simulink model "fuzzy_uirs"  (R2022a)
settings: Solver=FixedStepAuto  StartTime=0.0  StopTime=17  FixedStep=0.01  RelTol=1e-3
undefined symbols (not defined in the file): b, g, J, Ke, Kt, L, R
libraries: simulink_extras x9, slpidlib x3, fuzblock x3, simulink x1
settings Model: Creator=ngovi  LastModifiedBy=ngovi

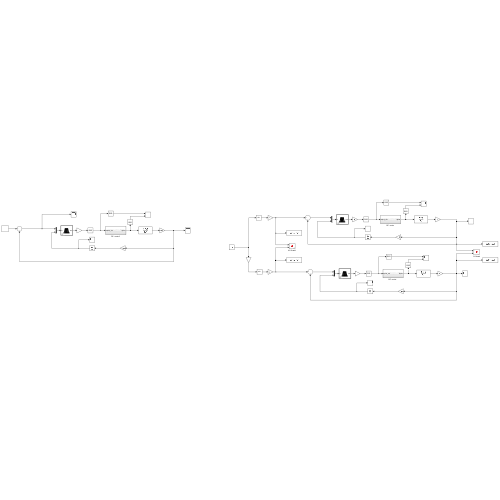
[thumbnail: Simulink's stored preview of the top-level diagram]
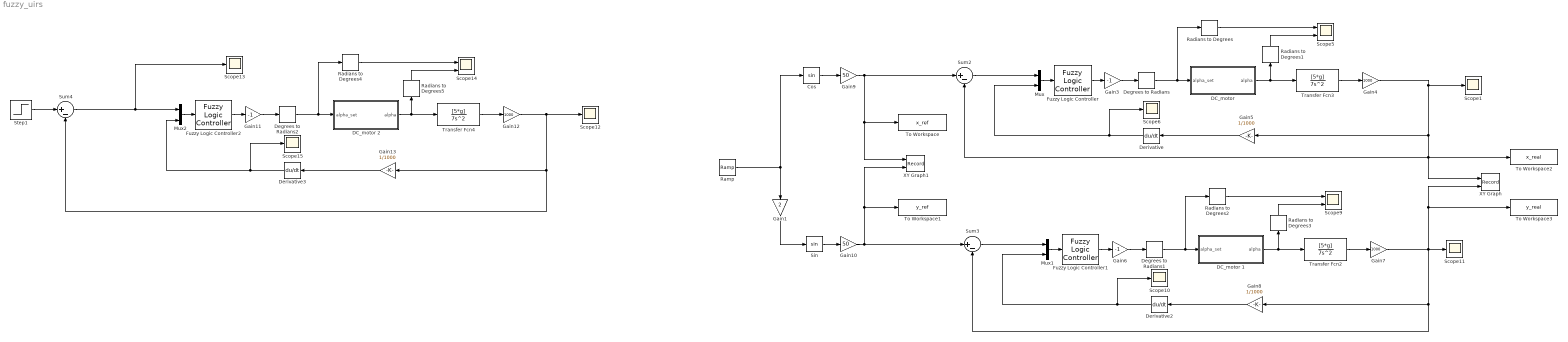
== system fuzzy_uirs ==
  Cos : Trigonometry
  "DC_motor " : Subsystem
  DC_motor 1 : Subsystem
  DC_motor 2 : Subsystem
  Degrees to Radians : simulink_extras/Transformations/Degrees to Radians
  Degrees to Radians1 : simulink_extras/Transformations/Degrees to Radians
  Degrees to Radians2 : simulink_extras/Transformations/Degrees to Radians
  Derivative : Derivative
  Derivative2 : Derivative
  Derivative3 : Derivative
  Fuzzy Logic Controller : fuzblock/Fuzzy Logic  Controller  FIS=logic3_3  OutputSampleNumber=101  DataType=double  FuzzifiedInputs=off  RuleFiringStrengths=off  RuleOutputs=off  AggregatedOutputs=off  SimulateUsing=Interpreted execution  OutOfRangeInputValueMessage=warning  NoRuleFiredMessage=warning  EmptyOutputFuzzySetMessage=warning
  Fuzzy Logic Controller1 : fuzblock/Fuzzy Logic  Controller  FIS=logic3_3  OutputSampleNumber=101  DataType=double  FuzzifiedInputs=off  RuleFiringStrengths=off  RuleOutputs=off  AggregatedOutputs=off  SimulateUsing=Interpreted execution  OutOfRangeInputValueMessage=warning  NoRuleFiredMessage=warning  EmptyOutputFuzzySetMessage=warning
  Fuzzy Logic Controller2 : fuzblock/Fuzzy Logic  Controller  FIS=logic3_3  OutputSampleNumber=101  DataType=double  FuzzifiedInputs=off  RuleFiringStrengths=off  RuleOutputs=off  AggregatedOutputs=off  SimulateUsing=Interpreted execution  OutOfRangeInputValueMessage=warning  NoRuleFiredMessage=warning  EmptyOutputFuzzySetMessage=warning
  Gain1 : Gain  Gain=2
  Gain10 : Gain  Gain=50
  Gain11 : Gain  Gain=-1
  Gain12 : Gain  Gain=1000
  Gain13 : Gain  Gain=1/1000
  Gain3 : Gain  Gain=-1
  Gain4 : Gain  Gain=1000
  Gain5 : Gain  Gain=1/1000
  Gain6 : Gain  Gain=-1
  Gain7 : Gain  Gain=1000
  Gain8 : Gain  Gain=1/1000
  Gain9 : Gain  Gain=50
  Mux : Mux  Inputs=2
  Mux1 : Mux  Inputs=2
  Mux2 : Mux  Inputs=2
  Radians to Degrees{,1..5} (6 alike) : simulink_extras/Transformations/Radians to Degrees
  Ramp : simulink/Sources/Ramp  slope=2*pi/15  start=0  InitialOutput=1
  Scope{1,6,10..13,15} (7 alike) : Scope
  Scope14 : Scope  NumInputPorts=2
  Scope5 : Scope  NumInputPorts=2
  Scope9 : Scope  NumInputPorts=2
  Sin : Trigonometry
  Step1 : Step  Time=0  After=50  SampleTime=0
  Sum2 : Sum  Inputs=|+-
  Sum3 : Sum  Inputs=|+-
  Sum4 : Sum  Inputs=|+-
  To Workspace : ToWorkspace  VariableName=x_ref  SampleTime=-1
  To Workspace1 : ToWorkspace  VariableName=y_ref  SampleTime=-1
  To Workspace2 : ToWorkspace  VariableName=x_real  SampleTime=-1
  To Workspace3 : ToWorkspace  VariableName=y_real  SampleTime=-1
  Transfer Fcn2 : TransferFcn  Numerator=[5*g]  Denominator=[7 0 0]
  Transfer Fcn3 : TransferFcn  Numerator=[5*g]  Denominator=[7 0 0]
  Transfer Fcn4 : TransferFcn  Numerator=[5*g]  Denominator=[7 0 0]
  XY Graph : Record  FileSettingsInternal="{\"entries\":[{\"content\":{\"excelSettings\":{\"content\":{},\"type\":\"Streamout.ExcelSettings\"}},\"type\":\"Streamout.FileSettingStorage\",\"uuid\":\"afb4c868-1969-4ea8-89d1-48caf8c4fd68\"}],\"packageUris\":[\"http://schema.mathworks.com/mf0/streamout_blocks/R2020a\"],\"version\":\"1.0\"}"  Layout=[1 1]  SignalsInternal="{\"entries\":[{\"content\":{\"signals\":[{\"content\":{\"blockPath\":[\"fuzzy_uirs/XY Graph\"],\"channel\":[],\"dimensions\":[1],\"domain\":\"fuzzy_uirs/XY Graph\",\"lineColor\":\"#a2142f\",\"plots\":[1],\"port\":1,\"sid\":[\"\"],\"signalID\":79152,\"signalName\":\"Gain4\"},\"type\":\"RecordBlkView.Signal\",\"uuid\":\"c0bbbc2e-870e-4cf8-b3f4-c9450fb1db15\"},{\"content\":{\"blockPath\":[\"fuzzy_uirs/XY Graph\"],\"channel\":[],\"dimensions\":[1],\"domain\":\"fuzzy_uirs/XY Graph\",\"lineColor\":\"#139fff\",\"plots\":[1],\"port\":2,\"sid\":[\"\"],\"signalID\":79156,\"signalName\":\"Gain7\"},\"type\":\"RecordBlkView.Signal\",\"uuid\":\"cc5d9cb4-a176-4346-b85d-aba7a873011e\"}]},\"type\":\"RecordBlkView.InputSignals\",\"uuid\":\"800058d3-d4f3-4397-acbe-427882f86b80\"}],\"packageUris\":[\"http://schema.mathworks.com/mf0/streamout_blocks/R2020a\"],\"version\":\"1.0\"}"  VisualizationBindings="{\"xyplotplugin\":{\"info\":[{\"series\":[{\"bindingParametersList\":[{\"parameter\":\"X-Axis\",\"signalID\":79152,\"signalName\":\"Gain4\"},{\"parameter\":\"Y-Axis\",\"signalID\":79156,\"signalName\":\"Gain7\"}],\"seriesID\":60483}],\"subplotID\":1}]}}"  CompatibilityTag=XY
  XY Graph1 : Record  FileSettingsInternal="{\"entries\":[{\"content\":{\"excelSettings\":{\"content\":{},\"type\":\"Streamout.ExcelSettings\"}},\"type\":\"Streamout.FileSettingStorage\",\"uuid\":\"2a686f37-4683-499c-9b28-704c226203bf\"}],\"packageUris\":[\"http://schema.mathworks.com/mf0/streamout_blocks/R2020a\"],\"version\":\"1.0\"}"  Layout=[1 1]  SignalsInternal="{\"entries\":[{\"content\":{\"signals\":[{\"content\":{\"blockPath\":[\"fuzzy_uirs/XY Graph1\"],\"channel\":[],\"dimensions\":[1],\"domain\":\"fuzzy_uirs/XY Graph1\",\"lineColor\":\"#a2142f\",\"plots\":[1],\"port\":1,\"sid\":[\"\"],\"signalID\":79160,\"signalName\":\"Gain9\"},\"type\":\"RecordBlkView.Signal\",\"uuid\":\"5bdc1996-2df4-4c65-8b97-25dc56d0c1d6\"},{\"content\":{\"blockPath\":[\"fuzzy_uirs/XY Graph1\"],\"channel\":[],\"dimensions\":[1],\"domain\":\"fuzzy_uirs/XY Graph1\",\"lineColor\":\"#139fff\",\"plots\":[1],\"port\":2,\"sid\":[\"\"],\"signalID\":79164,\"signalName\":\"Gain10\"},\"type\":\"RecordBlkView.Signal\",\"uuid\":\"afd1a10f-c0e4-4f62-abbc-f7fd10843523\"}]},\"type\":\"RecordBlkView.InputSignals\",\"uuid\":\"c62105ff-e949-4276-9948-db52a4e51b1c\"}],\"packageUris\":[\"http://schema.mathworks.com/mf0/streamout_blocks/R2020a\"],\"version\":\"1.0\"}"  VisualizationBindings="{\"xyplotplugin\":{\"info\":[{\"series\":[{\"bindingParametersList\":[{\"parameter\":\"X-Axis\",\"signalID\":79160,\"signalName\":\"Gain9\"},{\"parameter\":\"Y-Axis\",\"signalID\":79164,\"signalName\":\"Gain10\"}],\"seriesID\":17296}],\"subplotID\":1}]}}"  CompatibilityTag=XY
  wires:
  Fuzzy Logic Controller/1 -> Gain3/1
  Sum2/1 -> Mux/1
  "DC_motor "/1(alpha) -> Transfer Fcn3/1, Radians to Degrees1/1
  Mux/1 -> Fuzzy Logic Controller/1
  Derivative/1 -> Mux/2, Scope6/1
  Gain3/1 -> Degrees to Radians/1
  Degrees to Radians/1 -> Radians to Degrees/1, "DC_motor "/1(alpha_set)
  Transfer Fcn3/1 -> Gain4/1
  Gain4/1 -> Gain5/1, Sum2/2, XY Graph/1, To Workspace2/1, Scope1/1
  Gain5/1 -> Derivative/1
  Radians to Degrees/1 -> Scope5/1
  Radians to Degrees1/1 -> Scope5/2
  Radians to Degrees3/1 -> Scope9/2
  Radians to Degrees2/1 -> Scope9/1
  Gain8/1 -> Derivative2/1
  Gain7/1 -> Gain8/1, Sum3/2, To Workspace3/1, XY Graph/2, Scope11/1
  Transfer Fcn2/1 -> Gain7/1
  Degrees to Radians1/1 -> DC_motor 1/1(alpha_set), Radians to Degrees2/1
  Gain6/1 -> Degrees to Radians1/1
  Derivative2/1 -> Scope10/1, Mux1/2
  Mux1/1 -> Fuzzy Logic Controller1/1
  DC_motor 1/1(alpha) -> Radians to Degrees3/1, Transfer Fcn2/1
  Sum3/1 -> Mux1/1
  Sin/1 -> Gain10/1
  Fuzzy Logic Controller1/1 -> Gain6/1
  Ramp/1 -> Cos/1, Gain1/1
  Gain9/1 -> To Workspace/1, XY Graph1/1, Sum2/1
  Gain10/1 -> To Workspace1/1, XY Graph1/2, Sum3/1
  Step1/1 -> Sum4/1
  Radians to Degrees5/1 -> Scope14/2
  Radians to Degrees4/1 -> Scope14/1
  Gain13/1 -> Derivative3/1
  Gain12/1 -> Scope12/1, Gain13/1, Sum4/2
  Transfer Fcn4/1 -> Gain12/1
  Degrees to Radians2/1 -> DC_motor 2/1(alpha_set), Radians to Degrees4/1
  Gain11/1 -> Degrees to Radians2/1
  Derivative3/1 -> Mux2/2, Scope15/1
  Mux2/1 -> Fuzzy Logic Controller2/1
  Sum4/1 -> Scope13/1, Mux2/1
  Fuzzy Logic Controller2/1 -> Gain11/1
  DC_motor 2/1(alpha) -> Radians to Degrees5/1, Transfer Fcn4/1
  Cos/1 -> Gain9/1
  Gain1/1 -> Sin/1

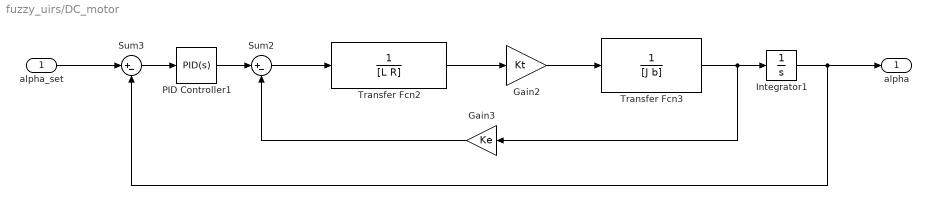
== system fuzzy_uirs/DC_motor  ==
  alpha_set : Inport
  Gain2 : Gain  Gain=Kt
  Gain3 : Gain  Gain=Ke
  Integrator1 : Integrator
  PID Controller1 : slpidlib/PID Controller  Controller=PID  Form=Parallel  TimeDomain=Continuous-time  UseExternalTs=off  SampleTime=-1  IntegratorMethod=Forward Euler  FilterMethod=Forward Euler  ControllerParametersSource=internal  P=0.045  I=0.0012  UseKiTs=off  D=0  N=100  UseFilter=on  TunerSelectOption=Transfer Function Based (PID Tuner App)  InitialConditionSource=internal  InitialConditionForIntegrator=0  InitialConditionForFilter=0  DifferentiatorICPrevScaledInput=0  ExternalReset=none  TrackingMode=off  Kt=1  LimitOutput=off  SatLimitsSource=internal  UpperSaturationLimit=inf  LowerSaturationLimit=-inf  LinearizeAsGain=on  AntiWindupMode=none  Kb=1  POutMin=[]  POutMax=[]  IOutMin=[]  IOutMax=[]  DOutMin=[]  DOutMax=[]  NOutMin=[]  NOutMax=[]  SumOutMin=[]  SumOutMax=[]  SaturationOutMin=[]  SaturationOutMax=[]  PParamMin=[]  PParamMax=[]  IParamMin=[]  IParamMax=[]  DParamMin=[]  DParamMax=[]  NParamMin=[]  NParamMax=[]  KbParamMin=[]  KbParamMax=[]  KtParamMin=[]  KtParamMax=[]  KbOutMin=[]  KbOutMax=[]  KtOutMin=[]  KtOutMax=[]  IntegratorOutMin=[]  IntegratorOutMax=[]  FilterOutMin=[]  FilterOutMax=[]  SumI1OutMin=[]  SumI1OutMax=[]  SumI2OutMin=[]  SumI2OutMax=[]  SumI3OutMin=[]  SumI3OutMax=[]  SumI4OutMin=[]  SumI4OutMax=[]  SumDOutMin=[]  SumDOutMax=[]  DifferentiatorOutMin=[]  DifferentiatorOutMax=[]  FilterDiffOutCoefMin=[]  FilterDiffOutCoefMax=[]  ReciprocalOutMin=[]  ReciprocalOutMax=[]  SumDenOutMin=[]  SumDenOutMax=[]  SumNumOutMin=[]  SumNumOutMax=[]  DivideOutMin=[]  DivideOutMax=[]  UdiffTsProdOutMin=[]  UdiffTsProdOutMax=[]  NTsProdOutMin=[]  NTsProdOutMax=[]  UintegralTsProdOutMin=[]  UintegralTsProdOutMax=[]  UngainTsProdOutMin=[]  UngainTsProdOutMax=[]  IntegratorContinuousStateAttributes=''  IntegratorStateMustResolveToSignalObject=off  IntegratorRTWStateStorageClass=Auto  FilterContinuousStateAttributes=''  FilterStateMustResolveToSignalObject=off  FilterRTWStateStorageClass=Auto  ParallelPVariant=InternalParameters  IdealPVariant=Disabled  IVariant=InternalParameters  DVariant=InternalParameters  IntegratorVariant=Continuous  SatVariant=Disabled  AWVariant=Passthrough  PCopyVariant=Disabled  TRVariant=Disabled  FdbkBlocksVariant=Forward  IdealPFdbkVariant=Disabled  SatFdbkVariant=Disabled  DerivativeFilterVariant=ContFilter  NVariant=InternalParameters  NCopyVariant=Disabled  FilterICVariant=InternalICsFilter  IntegratorICVariant=InternalICs  ExternalResetVariant=Disabled  TRSumVariant=Passthrough  SumFdbkVariant=Disabled  SumVariant=Sum_PID  TsampFilterVariant=InternalTs  TsampNgainVariant=Passthrough  TsampIntegralVariant=Passthrough  ExternalSaturationOutDataTypeStr=Inherit: Same as second input  aMode=0
  Sum2 : Sum  Inputs=|+-
  Sum3 : Sum  Inputs=|+-
  Transfer Fcn2 : TransferFcn  Denominator=[L R]
  Transfer Fcn3 : TransferFcn  Denominator=[J b]
  alpha : Outport
  wires:
  Transfer Fcn3/1 -> Integrator1/1, Gain3/1
  Transfer Fcn2/1 -> Gain2/1
  PID Controller1/1 -> Sum2/1
  Sum3/1 -> PID Controller1/1
  Gain2/1 -> Transfer Fcn3/1
  Integrator1/1 -> alpha/1, Sum3/2
  Gain3/1 -> Sum2/2
  Sum2/1 -> Transfer Fcn2/1
  alpha_set/1 -> Sum3/1

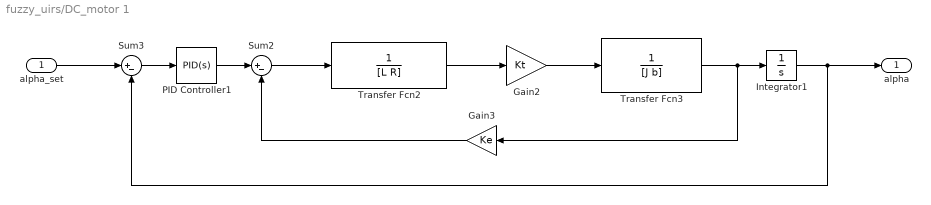
== system fuzzy_uirs/DC_motor 1 ==
  alpha_set : Inport
  Gain2 : Gain  Gain=Kt
  Gain3 : Gain  Gain=Ke
  Integrator1 : Integrator
  PID Controller1 : slpidlib/PID Controller  Controller=PID  Form=Parallel  TimeDomain=Continuous-time  UseExternalTs=off  SampleTime=-1  IntegratorMethod=Forward Euler  FilterMethod=Forward Euler  ControllerParametersSource=internal  P=0.045  I=0.0012  UseKiTs=off  D=0  N=100  UseFilter=on  TunerSelectOption=Transfer Function Based (PID Tuner App)  InitialConditionSource=internal  InitialConditionForIntegrator=0  InitialConditionForFilter=0  DifferentiatorICPrevScaledInput=0  ExternalReset=none  TrackingMode=off  Kt=1  LimitOutput=off  SatLimitsSource=internal  UpperSaturationLimit=inf  LowerSaturationLimit=-inf  LinearizeAsGain=on  AntiWindupMode=none  Kb=1  POutMin=[]  POutMax=[]  IOutMin=[]  IOutMax=[]  DOutMin=[]  DOutMax=[]  NOutMin=[]  NOutMax=[]  SumOutMin=[]  SumOutMax=[]  SaturationOutMin=[]  SaturationOutMax=[]  PParamMin=[]  PParamMax=[]  IParamMin=[]  IParamMax=[]  DParamMin=[]  DParamMax=[]  NParamMin=[]  NParamMax=[]  KbParamMin=[]  KbParamMax=[]  KtParamMin=[]  KtParamMax=[]  KbOutMin=[]  KbOutMax=[]  KtOutMin=[]  KtOutMax=[]  IntegratorOutMin=[]  IntegratorOutMax=[]  FilterOutMin=[]  FilterOutMax=[]  SumI1OutMin=[]  SumI1OutMax=[]  SumI2OutMin=[]  SumI2OutMax=[]  SumI3OutMin=[]  SumI3OutMax=[]  SumI4OutMin=[]  SumI4OutMax=[]  SumDOutMin=[]  SumDOutMax=[]  DifferentiatorOutMin=[]  DifferentiatorOutMax=[]  FilterDiffOutCoefMin=[]  FilterDiffOutCoefMax=[]  ReciprocalOutMin=[]  ReciprocalOutMax=[]  SumDenOutMin=[]  SumDenOutMax=[]  SumNumOutMin=[]  SumNumOutMax=[]  DivideOutMin=[]  DivideOutMax=[]  UdiffTsProdOutMin=[]  UdiffTsProdOutMax=[]  NTsProdOutMin=[]  NTsProdOutMax=[]  UintegralTsProdOutMin=[]  UintegralTsProdOutMax=[]  UngainTsProdOutMin=[]  UngainTsProdOutMax=[]  IntegratorContinuousStateAttributes=''  IntegratorStateMustResolveToSignalObject=off  IntegratorRTWStateStorageClass=Auto  FilterContinuousStateAttributes=''  FilterStateMustResolveToSignalObject=off  FilterRTWStateStorageClass=Auto  ParallelPVariant=InternalParameters  IdealPVariant=Disabled  IVariant=InternalParameters  DVariant=InternalParameters  IntegratorVariant=Continuous  SatVariant=Disabled  AWVariant=Passthrough  PCopyVariant=Disabled  TRVariant=Disabled  FdbkBlocksVariant=Forward  IdealPFdbkVariant=Disabled  SatFdbkVariant=Disabled  DerivativeFilterVariant=ContFilter  NVariant=InternalParameters  NCopyVariant=Disabled  FilterICVariant=InternalICsFilter  IntegratorICVariant=InternalICs  ExternalResetVariant=Disabled  TRSumVariant=Passthrough  SumFdbkVariant=Disabled  SumVariant=Sum_PID  TsampFilterVariant=InternalTs  TsampNgainVariant=Passthrough  TsampIntegralVariant=Passthrough  ExternalSaturationOutDataTypeStr=Inherit: Same as second input  aMode=0
  Sum2 : Sum  Inputs=|+-
  Sum3 : Sum  Inputs=|+-
  Transfer Fcn2 : TransferFcn  Denominator=[L R]
  Transfer Fcn3 : TransferFcn  Denominator=[J b]
  alpha : Outport
  wires:
  alpha_set/1 -> Sum3/1
  Sum2/1 -> Transfer Fcn2/1
  Gain3/1 -> Sum2/2
  Integrator1/1 -> Sum3/2, alpha/1
  Gain2/1 -> Transfer Fcn3/1
  Sum3/1 -> PID Controller1/1
  PID Controller1/1 -> Sum2/1
  Transfer Fcn2/1 -> Gain2/1
  Transfer Fcn3/1 -> Gain3/1, Integrator1/1

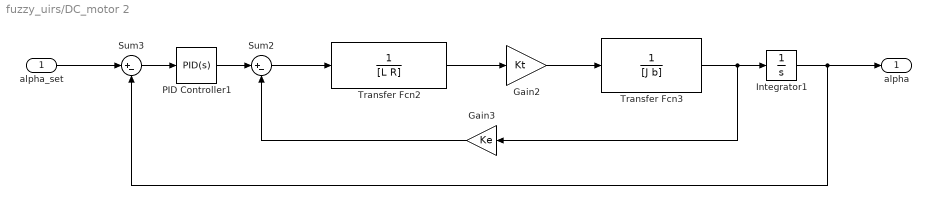
== system fuzzy_uirs/DC_motor 2 ==
  alpha_set : Inport
  Gain2 : Gain  Gain=Kt
  Gain3 : Gain  Gain=Ke
  Integrator1 : Integrator
  PID Controller1 : slpidlib/PID Controller  Controller=PID  Form=Parallel  TimeDomain=Continuous-time  UseExternalTs=off  SampleTime=-1  IntegratorMethod=Forward Euler  FilterMethod=Forward Euler  ControllerParametersSource=internal  P=0.045  I=0.0012  UseKiTs=off  D=0  N=100  UseFilter=on  TunerSelectOption=Transfer Function Based (PID Tuner App)  InitialConditionSource=internal  InitialConditionForIntegrator=0  InitialConditionForFilter=0  DifferentiatorICPrevScaledInput=0  ExternalReset=none  TrackingMode=off  Kt=1  LimitOutput=off  SatLimitsSource=internal  UpperSaturationLimit=inf  LowerSaturationLimit=-inf  LinearizeAsGain=on  AntiWindupMode=none  Kb=1  POutMin=[]  POutMax=[]  IOutMin=[]  IOutMax=[]  DOutMin=[]  DOutMax=[]  NOutMin=[]  NOutMax=[]  SumOutMin=[]  SumOutMax=[]  SaturationOutMin=[]  SaturationOutMax=[]  PParamMin=[]  PParamMax=[]  IParamMin=[]  IParamMax=[]  DParamMin=[]  DParamMax=[]  NParamMin=[]  NParamMax=[]  KbParamMin=[]  KbParamMax=[]  KtParamMin=[]  KtParamMax=[]  KbOutMin=[]  KbOutMax=[]  KtOutMin=[]  KtOutMax=[]  IntegratorOutMin=[]  IntegratorOutMax=[]  FilterOutMin=[]  FilterOutMax=[]  SumI1OutMin=[]  SumI1OutMax=[]  SumI2OutMin=[]  SumI2OutMax=[]  SumI3OutMin=[]  SumI3OutMax=[]  SumI4OutMin=[]  SumI4OutMax=[]  SumDOutMin=[]  SumDOutMax=[]  DifferentiatorOutMin=[]  DifferentiatorOutMax=[]  FilterDiffOutCoefMin=[]  FilterDiffOutCoefMax=[]  ReciprocalOutMin=[]  ReciprocalOutMax=[]  SumDenOutMin=[]  SumDenOutMax=[]  SumNumOutMin=[]  SumNumOutMax=[]  DivideOutMin=[]  DivideOutMax=[]  UdiffTsProdOutMin=[]  UdiffTsProdOutMax=[]  NTsProdOutMin=[]  NTsProdOutMax=[]  UintegralTsProdOutMin=[]  UintegralTsProdOutMax=[]  UngainTsProdOutMin=[]  UngainTsProdOutMax=[]  IntegratorContinuousStateAttributes=''  IntegratorStateMustResolveToSignalObject=off  IntegratorRTWStateStorageClass=Auto  FilterContinuousStateAttributes=''  FilterStateMustResolveToSignalObject=off  FilterRTWStateStorageClass=Auto  ParallelPVariant=InternalParameters  IdealPVariant=Disabled  IVariant=InternalParameters  DVariant=InternalParameters  IntegratorVariant=Continuous  SatVariant=Disabled  AWVariant=Passthrough  PCopyVariant=Disabled  TRVariant=Disabled  FdbkBlocksVariant=Forward  IdealPFdbkVariant=Disabled  SatFdbkVariant=Disabled  DerivativeFilterVariant=ContFilter  NVariant=InternalParameters  NCopyVariant=Disabled  FilterICVariant=InternalICsFilter  IntegratorICVariant=InternalICs  ExternalResetVariant=Disabled  TRSumVariant=Passthrough  SumFdbkVariant=Disabled  SumVariant=Sum_PID  TsampFilterVariant=InternalTs  TsampNgainVariant=Passthrough  TsampIntegralVariant=Passthrough  ExternalSaturationOutDataTypeStr=Inherit: Same as second input  aMode=0
  Sum2 : Sum  Inputs=|+-
  Sum3 : Sum  Inputs=|+-
  Transfer Fcn2 : TransferFcn  Denominator=[L R]
  Transfer Fcn3 : TransferFcn  Denominator=[J b]
  alpha : Outport
  wires:
  alpha_set/1 -> Sum3/1
  Sum2/1 -> Transfer Fcn2/1
  Gain3/1 -> Sum2/2
  Integrator1/1 -> Sum3/2, alpha/1
  Gain2/1 -> Transfer Fcn3/1
  Sum3/1 -> PID Controller1/1
  PID Controller1/1 -> Sum2/1
  Transfer Fcn2/1 -> Gain2/1
  Transfer Fcn3/1 -> Gain3/1, Integrator1/1
